simulink model "SOC_SOP_SOE_Estimator_prev"  (R2022b)
settings: Solver=VariableStepAuto  StartTime=0.0  StopTime=10.0  RelTol=1e-3
values from neighbouring files (symbols this model uses):
  C1_Matrix = 422.2404285437554 832.53586872460221 593.83691968900087 100.00008052662714 100.0001060028228 100.00352207851405 573.68336177620586 595.79755617901333 100.00046144734698 100.00010895024188 100.00001099617816 100.00006837618552 691.48671856868566 2134.4373901996432 816.34740544716044 806.77260368332577 100.0467458146305 598.37385117856434 100.00076319616421 859.37820132571676 896.36317538528124 1484    [Estimators_Dictionary.sldd]
  C2_Matrix = 1869.0199173311939 2837.236592228945 2101.4831882408225 1494.0038217573228 1387.7964069745447 1517.4535489073862 2616.2107406796117 2389.8139537375896 1452.8919060078656 1228.7968116693385 1198.856242336575 1171.693964913431 6721.2581904188037 1000.0000000113553 9531.2637756330168 5076.9051378834283 1199.7174655557417 1384.2253611332994 1210.6925685743531 5536.2724577262752 3310.8601470778594 4071    [Estimators_Dictionary.sldd]
  C3_Matrix = 10000.000413012229 10000.437423538908 10000.000000002954 999999.99836905929 999999.99999998079 10000.000000003132 10006.050761940998 10005.494579451251 10000.00000000291 999999.999999997 999999.99999999709 999999.99999999709 10000.206379215075 999999.999999997 10000.0000221827 10000.008256352026 25318.524233270309 999999.99999986857 999999.99999999709 33014.106269942291 10000.002694208375 10000.00    [Estimators_Dictionary.sldd]
  Capacity_Vec : value not decoded    [Estimators_Dictionary.sldd]
  Current_Vec : value not decoded    [Estimators_Dictionary.sldd]
  Initial_Covariance : value not decoded    [Estimators_Dictionary.sldd]
  L_SOP = 10.0    [Estimators_Dictionary.sldd]
  MaxChargeCurrent = -4.5    [Estimators_Dictionary.sldd]
  MaxDischargeCurrent = 13.5    [Estimators_Dictionary.sldd]
  Measurement_Noise_Covariance : value not decoded    [Estimators_Dictionary.sldd]
  NumberSt = 4.0    [Estimators_Dictionary.sldd]
  NumModules = 1.0    [Global_Parameters.sldd]
  NumParallel = 30.0    [Global_Parameters.sldd]
  NumSeries = 24.0    [Global_Parameters.sldd]
  OCV_25 = 2.499931353 2.660173565 2.770290801 2.849668545 2.910864288 2.961377818 3.004426237 3.041700228 3.074206823 3.103359053 3.130289569 3.156365364 3.182882947 3.209913924 3.23738746 3.264399583 3.29032752 3.314243172 3.336274664 3.356562434 3.375508383 3.393471938 3.410420203 3.425459892 3.444565547 3.460488492 3.470240307 3.477937034 3.484868617 3.491737023 3.49969269 3.561668176 3.613859701 3.66247    [Estimators_Dictionary.sldd]
  OCV_Matrix = 2.499880511 2.757887899 2.885852779 2.958886734 3.012482188 3.054053996 3.088246035 3.118484978 3.146762309 3.174638012 3.202260862 3.229457219 3.25550064 3.2799103 3.302460407 3.323174742 3.342372966 3.36043721 3.377577579 3.393845327 3.409287366 3.424345095 3.438835902 3.451705646 3.462748292 3.471979517 3.479948585 3.487316883 3.494719929 3.502771519 3.512228835 3.565792216 3.611361646 3.654868    [Estimators_Dictionary.sldd]
  Process_Noise_Covariance : value not decoded    [Estimators_Dictionary.sldd]
  R0_Matrix = 0.078 0.065280058 0.057635214 0.051424984 0.047235164 0.045274346 0.044600944 0.044414272 0.043883424 0.043849968 0.043505816 0.043376214 0.042951864 0.042984622 0.04246783 0.042081824 0.04225864 0.042254038 0.042812396 0.044036376 0.046360714 0.04 0.027933632 0.02654818 0.0250776 0.024521118 0.02407035 0.023664778 0.023539386 0.023690548 0.023919438 0.023613406 0.023919438 0.023462652 0.023664778    [Estimators_Dictionary.sldd]
  R1_Matrix = 0.0088889584036008756 0.011132450225251986 0.0047020868736295475 0.0038328697373028187 0.0040332105595120874 0.0042459601469587993 0.0079556549223052976 0.0077202921614856973 0.0042458367238840319 0.0037380352668936129 0.0039024749524341363 0.0039171117297991413 0.011740686313090084 0.019999999846677257 0.016223479832535404 0.012377879169958896 0.0036112899599241629 0.0044757607076317636 0.0037164    [Estimators_Dictionary.sldd]
  R2_Matrix = 0.019999839352755313 0.018530158856651584 0.019999999999991039 0.019999999999999653 0.019094577060873957 0.019999999999999653 0.017574853989291029 0.018122428670813852 0.01999999999999965 0.017630542321676212 0.018068015705526037 0.018465022507068402 0.005950765066923343 0.0091611667859414717 0.0094260137994600333 0.010899029961443308 0.019999999999999508 0.019999999993878602 0.018482036338747981    [Estimators_Dictionary.sldd]
  R3_Matrix = 0.011000556558775975 0.0057135937221727282 0.0099840161409517954 0.0010000000000003474 0.0010000000000003476 0.0011277504341113288 0.002355571622354306 0.0020545810808267474 0.0011567518791196808 0.00100000000000035 0.0010000000000003485 0.0010000000000003491 0.0045246675537304517 0.0010000000004847253 0.0058172911331956572 0.0046897007611929825 0.003722001496194627 0.0010000000001368907 0.0010000    [Estimators_Dictionary.sldd]
  RC_SOC_Vec : value not decoded    [Estimators_Dictionary.sldd]
  SOC_Max = 1.0    [Estimators_Dictionary.sldd]
  SOC_Min = 0.0    [Estimators_Dictionary.sldd]
  SOC_Vec1 : value not decoded    [Estimators_Dictionary.sldd]
  SOC_Vec2 = 0.0426283206867574 0.0904968112442659 0.138364796472968 0.186232899174877 0.234100725864356 0.281969477464203 0.329837548126425 0.37770754411239 0.425577249630283 0.473445315109007 0.52131352299741 0.569182352268543 0.617052114517866 0.664920478266386 0.712789145362285 0.760657112801272 0.808525199586941 0.856393952315712 0.904262172378725 0.952130333891273 1.0    [Estimators_Dictionary.sldd]
  SOH_Vec : value not decoded    [Estimators_Dictionary.sldd]
  Temperature_Vec : value not decoded    [Estimators_Dictionary.sldd]
  Ts = 0.01    [Global_Parameters.sldd]
  Ts_SOP = 15.0    [Estimators_Dictionary.sldd]
  V1_Max = 0.01    [Estimators_Dictionary.sldd]
  V1_Min = -0.01    [Estimators_Dictionary.sldd]
  V2_Max = 0.01    [Estimators_Dictionary.sldd]
  V2_Min = -0.01    [Estimators_Dictionary.sldd]
  V3_Max = 0.01    [Estimators_Dictionary.sldd]
  V3_Min = -0.01    [Estimators_Dictionary.sldd]
  Vmax = 4.1    [Global_Parameters.sldd]
  Vmin = 3.0    [Global_Parameters.sldd]
settings Model: DataDictionary=Estimators_Dictionary.sldd  Creator=japerez  LastModifiedBy=CMARTINEZ
settings DebuggingCC: ParameterPrecisionLossMsg=none

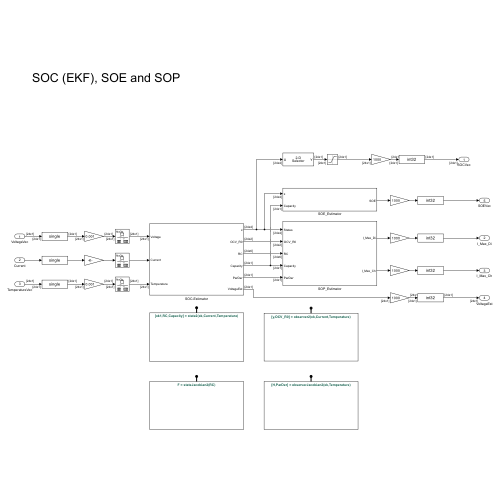
[thumbnail: Simulink's stored preview of the top-level diagram]
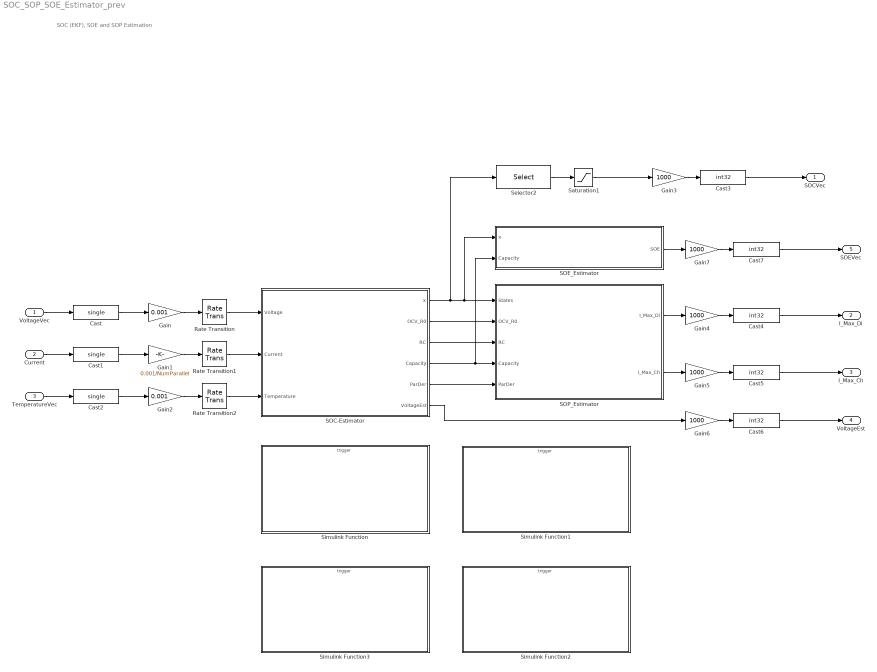
== system SOC_SOP_SOE_Estimator_prev ==
  note: SOC (EKF), SOE and SOP Estimation
  VoltageVec : Inport  OutDataTypeStr=int32  PortDimensions=[NumSeries*NumModules,1]
  Current : Inport  Port=2  OutDataTypeStr=int32  PortDimensions=1
  TemperatureVec : Inport  Port=3  OutDataTypeStr=int32  PortDimensions=[NumSeries*NumModules,1]
  Cast : DataTypeConversion  OutDataTypeStr=single  SaturateOnIntegerOverflow=off  RndMeth=Floor
  Cast1 : DataTypeConversion  OutDataTypeStr=single  SaturateOnIntegerOverflow=off  RndMeth=Floor
  Cast2 : DataTypeConversion  OutDataTypeStr=single  SaturateOnIntegerOverflow=off  RndMeth=Floor
  Cast{3..7} (5 alike) : DataTypeConversion  OutDataTypeStr=int32  SaturateOnIntegerOverflow=off  RndMeth=Floor
  Gain : Gain  Gain=0.001
  Gain1 : Gain  Gain=0.001/NumParallel
  Gain2 : Gain  Gain=0.001
  Gain{3..7} (5 alike) : Gain  Gain=1000
  Rate Transition : RateTransition  Integrity=off  OutPortSampleTime=Ts
  Rate Transition1 : RateTransition  Integrity=off  OutPortSampleTime=Ts
  Rate Transition2 : RateTransition  Integrity=off  OutPortSampleTime=Ts
  SOC-Estimator : Subsystem
  SOE_Estimator : Subsystem
  SOP_Estimator : Subsystem
  Saturation1 : Saturate  UpperLimit=1  LowerLimit=0
  Selector2 : Selector  NumberOfDimensions=2  InputPortWidth=24  IndexOptions=Select all,Index vector (dialog)  Indices=1,1  OutputSizes=1,1
  Simulink Function : Subsystem  TreatAsAtomicUnit=on
  Simulink Function1 : Subsystem  TreatAsAtomicUnit=on
  Simulink Function2 : Subsystem  TreatAsAtomicUnit=on
  Simulink Function3 : Subsystem  TreatAsAtomicUnit=on
  SOCVec : Outport  OutDataTypeStr=int32  PortDimensions=[NumSeries*NumModules,1]
  I_Max_Di : Outport  Port=2  OutDataTypeStr=int32  PortDimensions=1
  I_Max_Ch : Outport  Port=3  OutDataTypeStr=int32  PortDimensions=1
  VoltageEst : Outport  Port=4  OutDataTypeStr=int32  PortDimensions=[NumSeries*NumModules,1]
  SOEVec : Outport  Port=5
  wires:
  Gain/1 -> Rate Transition/1
  Rate Transition2/1 -> SOC-Estimator/3(Temperature)
  Gain1/1 -> Rate Transition1/1
  Selector2/1 -> Saturation1/1
  VoltageVec/1 -> Cast/1
  Current/1 -> Cast1/1
  TemperatureVec/1 -> Cast2/1
  Cast/1 -> Gain/1
  Cast1/1 -> Gain1/1
  Cast2/1 -> Gain2/1
  Gain2/1 -> Rate Transition2/1
  Gain3/1 -> Cast3/1
  Saturation1/1 -> Gain3/1
  SOC-Estimator/1(x) -> SOE_Estimator/1(x), SOP_Estimator/1(States), Selector2/1
  SOC-Estimator/2(OCV_R0) -> SOP_Estimator/2(OCV_R0)
  SOC-Estimator/3(RC) -> SOP_Estimator/3(RC)
  SOC-Estimator/4(Capacity) -> SOE_Estimator/2(Capacity), SOP_Estimator/4(Capacity)
  SOC-Estimator/5(ParDer) -> SOP_Estimator/5(ParDer)
  Gain4/1 -> Cast4/1
  SOP_Estimator/1(I_Max_Di) -> Gain4/1
  Gain5/1 -> Cast5/1
  SOP_Estimator/2(I_Max_Ch) -> Gain5/1
  Gain6/1 -> Cast6/1
  SOC-Estimator/6(VoltageEst) -> Gain6/1
  Rate Transition1/1 -> SOC-Estimator/2(Current)
  Rate Transition/1 -> SOC-Estimator/1(Voltage)
  Cast3/1 -> SOCVec/1
  Cast4/1 -> I_Max_Di/1
  Cast5/1 -> I_Max_Ch/1
  Cast6/1 -> VoltageEst/1
  SOE_Estimator/1(SOE) -> Gain7/1
  Gain7/1 -> Cast7/1
  Cast7/1 -> SOEVec/1

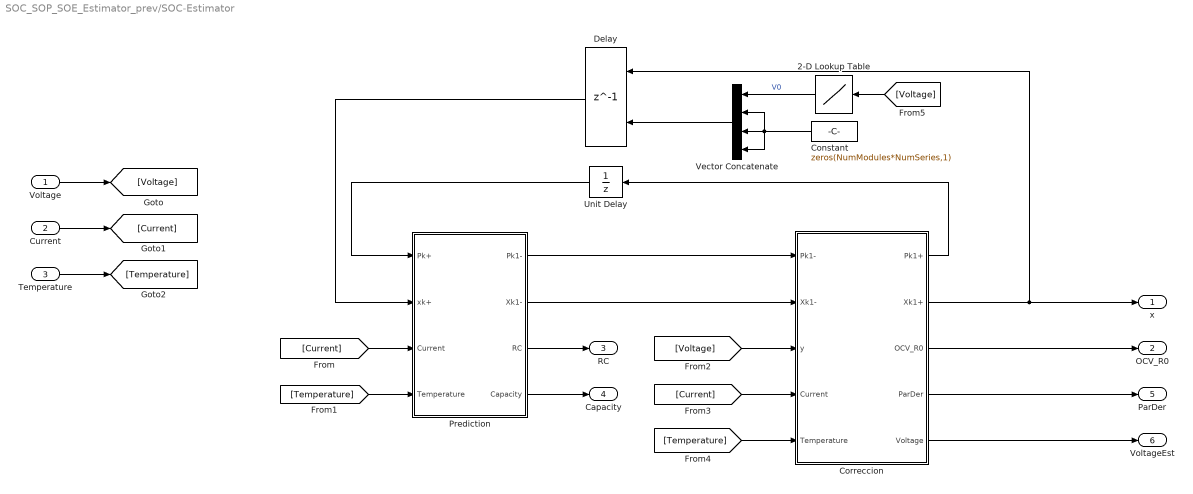
== system SOC_SOP_SOE_Estimator_prev/SOC-Estimator ==
  Voltage : Inport
  Current : Inport  Port=2
  Temperature : Inport  Port=3
  2-D Lookup Table : Lookup_n-D  NumberOfTableDimensions=1  BreakpointsForDimension1=OCV_25  BreakpointsForDimension2=Temperature_Vec  BreakpointsForDimension3=SOH_Vec  Table=SOC_Vec1  ExtrapMethod=Clip  InternalRulePriority=Speed  RndMeth=Simplest
  Constant : Constant  Value=zeros(NumModules*NumSeries,1)  OutDataTypeStr=single
  Correccion : Subsystem
  Delay : Delay  DelayLength=1  InitialConditionSource=Input port
      settings: InputPortMap=u0,p4
  Prediction : Subsystem
  Unit Delay : UnitDelay  InitialCondition=Initial_Covariance.*ones(NumModules*NumSeries,NumberSt)  SampleTime=Ts  HasFrameUpgradeWarning=on
  Vector Concatenate : Concatenate  NumInputs=4  Mode=Multidimensional array  ConcatenateDimension=2
  x : Outport
  OCV_R0 : Outport  Port=2
  RC : Outport  Port=3
  Capacity : Outport  Port=4
  ParDer : Outport  Port=5
  VoltageEst : Outport  Port=6
  wires:
  [Current] -> Prediction/3(Current)
  [Temperature] -> Prediction/4(Temperature)
  Temperature/1 -> [Temperature]
  Correccion/1(Pk1+) -> Unit Delay/1
  Prediction/1(Pk1-) -> Correccion/1(Pk1-)
  Prediction/2(Xk1-) -> Correccion/2(Xk1-)
  Correccion/2(Xk1+) -> Delay/1, x/1
  [Voltage] -> Correccion/3(y)
  Voltage/1 -> [Voltage]
  Current/1 -> [Current]
  Unit Delay/1 -> Prediction/1(Pk+)
  [Temperature] -> Correccion/5(Temperature)
  [Current] -> Correccion/4(Current)
  Correccion/3(OCV_R0) -> OCV_R0/1
  Delay/1 -> Prediction/2(xk+)
  Prediction/3(RC) -> RC/1
  Prediction/4(Capacity) -> Capacity/1
  Correccion/4(ParDer) -> ParDer/1
  Correccion/5(Voltage) -> VoltageEst/1
  Constant/1 -> Vector Concatenate/2, Vector Concatenate/3, Vector Concatenate/4
  2-D Lookup Table/1 -> Vector Concatenate/1  "V0"
  Vector Concatenate/1 -> Delay/2
  [Voltage] -> 2-D Lookup Table/1

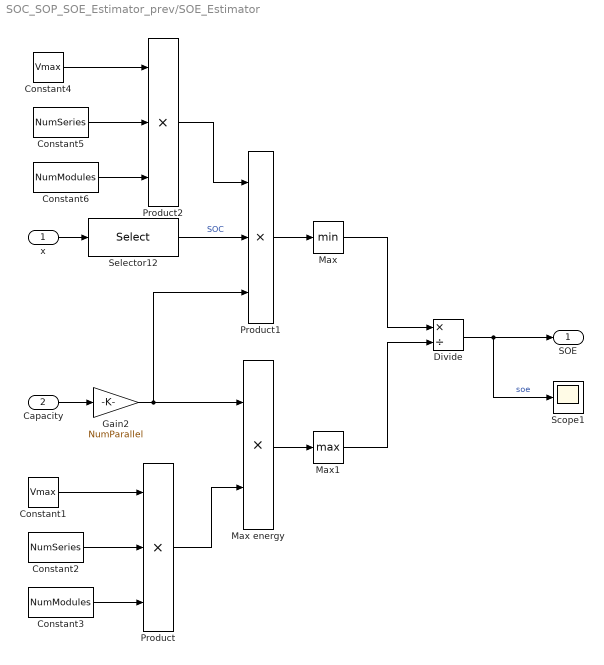
== system SOC_SOP_SOE_Estimator_prev/SOE_Estimator ==
  x : Inport
  Capacity : Inport  Port=2
  Constant1 : Constant  Value=Vmax
  Constant2 : Constant  Value=NumSeries
  Constant3 : Constant  Value=NumModules
  Constant4 : Constant  Value=Vmax
  Constant5 : Constant  Value=NumSeries
  Constant6 : Constant  Value=NumModules
  Divide : Product  Inputs=*/
  Gain2 : Gain  Gain=NumParallel
  Max : MinMax
  Max energy : Product
  Max1 : MinMax  Function=max
  Product : Product  Inputs=3
  Product1 : Product  Inputs=3
  Product2 : Product  Inputs=3
  Scope1 : Scope
  Selector12 : Selector  NumberOfDimensions=2  InputPortWidth=24  IndexOptions=Select all,Index vector (dialog)  Indices=1,1  OutputSizes=1,1
  SOE : Outport  OutDataTypeStr=single
  wires:
  x/1 -> Selector12/1
  Constant1/1 -> Product/1
  Constant2/1 -> Product/2
  Capacity/1 -> Gain2/1
  Product/1 -> Max energy/2
  Max/1 -> Divide/1
  Max1/1 -> Divide/2
  Divide/1 -> SOE/1, Scope1/1  "soe"
  Product1/1 -> Max/1
  Max energy/1 -> Max1/1
  Constant3/1 -> Product/3
  Selector12/1 -> Product1/2  "SOC"
  Constant6/1 -> Product2/3
  Constant5/1 -> Product2/2
  Constant4/1 -> Product2/1
  Product2/1 -> Product1/1
  Gain2/1 -> Product1/3, Max energy/1

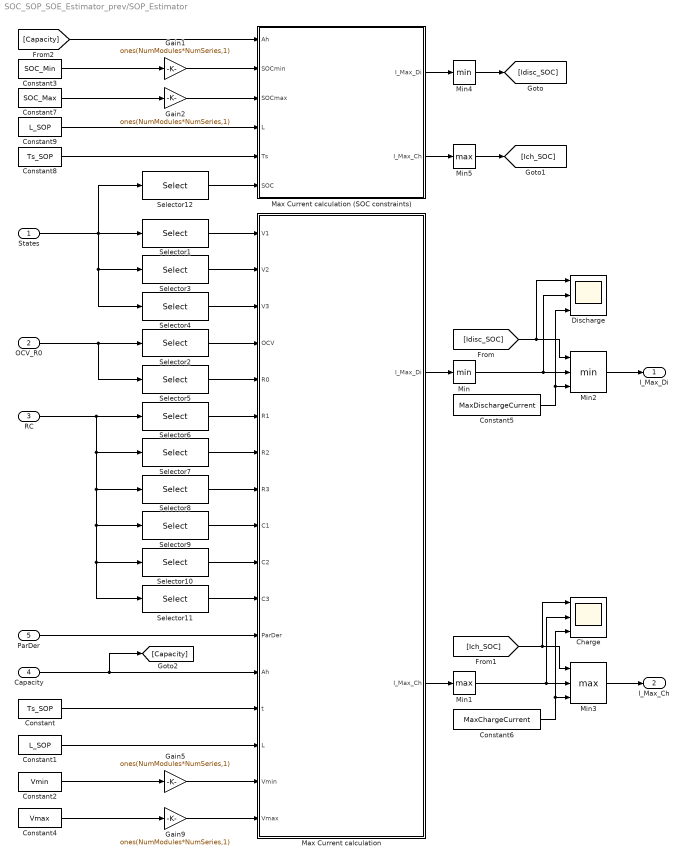
== system SOC_SOP_SOE_Estimator_prev/SOP_Estimator ==
  States : Inport  OutDataTypeStr=single  PortDimensions=[NumModules*NumSeries,NumberSt]
  OCV_R0 : Inport  Port=2  OutDataTypeStr=single  PortDimensions=[NumModules*NumSeries,2]
  RC : Inport  Port=3  OutDataTypeStr=single  PortDimensions=[NumModules*NumSeries,6]
  Capacity : Inport  Port=4  OutDataTypeStr=single  PortDimensions=[NumModules*NumSeries,1]
  ParDer : Inport  Port=5  OutDataTypeStr=single  PortDimensions=[NumModules*NumSeries,1]
  Charge : Scope  NumInputPorts=3
  Constant : Constant  Value=Ts_SOP
  Constant1 : Constant  Value=L_SOP
  Constant2 : Constant  Value=Vmin  OutDataTypeStr=single
  Constant3 : Constant  Value=SOC_Min  OutDataTypeStr=single
  Constant4 : Constant  Value=Vmax  OutDataTypeStr=single
  Constant5 : Constant  Value=MaxDischargeCurrent
  Constant6 : Constant  Value=MaxChargeCurrent
  Constant7 : Constant  Value=SOC_Max  OutDataTypeStr=single
  Constant8 : Constant  Value=Ts_SOP
  Constant9 : Constant  Value=L_SOP
  Discharge : Scope  NumInputPorts=3
  Gain{1..2,5,9} (4 alike) : Gain  Gain=ones(NumModules*NumSeries,1)  ParamDataTypeStr=single  OutDataTypeStr=single
  Max Current calculation : MATLAB Function  TreatAsAtomicUnit=on
  Max Current calculation (SOC constraints) : MATLAB Function  TreatAsAtomicUnit=on
  Min : MinMax
  Min1 : MinMax  Function=max
  Min2 : MinMax  Inputs=3
  Min3 : MinMax  Function=max  Inputs=3
  Min4 : MinMax
  Min5 : MinMax  Function=max
  Selector1 : Selector  NumberOfDimensions=2  InputPortWidth=24  IndexOptions=Select all,Index vector (dialog)  Indices=1,2  OutputSizes=1,1
  Selector10 : Selector  NumberOfDimensions=2  InputPortWidth=24  IndexOptions=Select all,Index vector (dialog)  Indices=1,5  OutputSizes=1,1
  Selector11 : Selector  NumberOfDimensions=2  InputPortWidth=24  IndexOptions=Select all,Index vector (dialog)  Indices=1,6  OutputSizes=1,1
  Selector12 : Selector  NumberOfDimensions=2  InputPortWidth=24  IndexOptions=Select all,Index vector (dialog)  Indices=1,1  OutputSizes=1,1
  Selector2 : Selector  NumberOfDimensions=2  InputPortWidth=24  IndexOptions=Select all,Index vector (dialog)  Indices=1,1  OutputSizes=1,1
  Selector3 : Selector  NumberOfDimensions=2  InputPortWidth=24  IndexOptions=Select all,Index vector (dialog)  Indices=1,3  OutputSizes=1,1
  Selector4 : Selector  NumberOfDimensions=2  InputPortWidth=24  IndexOptions=Select all,Index vector (dialog)  Indices=1,4  OutputSizes=1,1
  Selector5 : Selector  NumberOfDimensions=2  InputPortWidth=24  IndexOptions=Select all,Index vector (dialog)  Indices=1,2  OutputSizes=1,1
  Selector6 : Selector  NumberOfDimensions=2  InputPortWidth=24  IndexOptions=Select all,Index vector (dialog)  Indices=1,1  OutputSizes=1,1
  Selector7 : Selector  NumberOfDimensions=2  InputPortWidth=24  IndexOptions=Select all,Index vector (dialog)  Indices=1,2  OutputSizes=1,1
  Selector8 : Selector  NumberOfDimensions=2  InputPortWidth=24  IndexOptions=Select all,Index vector (dialog)  Indices=1,3  OutputSizes=1,1
  Selector9 : Selector  NumberOfDimensions=2  InputPortWidth=24  IndexOptions=Select all,Index vector (dialog)  Indices=1,4  OutputSizes=1,1
  I_Max_Di : Outport  OutDataTypeStr=single  PortDimensions=1
  I_Max_Ch : Outport  Port=2  OutDataTypeStr=single  PortDimensions=1
  wires:
  Selector1/1 -> Max Current calculation/1(V1)
  Selector5/1 -> Max Current calculation/5(R0)
  Constant2/1 -> Gain5/1
  Max Current calculation/2(I_Max_Ch) -> Min1/1
  Min2/1 -> I_Max_Di/1
  Max Current calculation/1(I_Max_Di) -> Min/1
  Constant4/1 -> Gain9/1
  OCV_R0/1 -> Selector5/1, Selector2/1
  Gain5/1 -> Max Current calculation/16(Vmin)
  Capacity/1 -> [Capacity], Max Current calculation/13(Ah)
  Selector3/1 -> Max Current calculation/2(V2)
  Min3/1 -> I_Max_Ch/1
  RC/1 -> Selector11/1, Selector10/1, Selector9/1, Selector8/1, Selector7/1, Selector6/1
  Selector2/1 -> Max Current calculation/4(OCV)
  Selector6/1 -> Max Current calculation/6(R1)
  Selector11/1 -> Max Current calculation/11(C3)
  Selector10/1 -> Max Current calculation/10(C2)
  Selector9/1 -> Max Current calculation/9(C1)
  ParDer/1 -> Max Current calculation/12(ParDer)
  Selector8/1 -> Max Current calculation/8(R3)
  Selector7/1 -> Max Current calculation/7(R2)
  Selector4/1 -> Max Current calculation/3(V3)
  Constant1/1 -> Max Current calculation/15(L)
  Gain9/1 -> Max Current calculation/17(Vmax)
  Constant3/1 -> Gain1/1
  States/1 -> Selector12/1, Selector4/1, Selector3/1, Selector1/1
  Constant7/1 -> Gain2/1
  Selector12/1 -> Max Current calculation (SOC constraints)/6(SOC)
  Gain2/1 -> Max Current calculation (SOC constraints)/3(SOCmax)
  Gain1/1 -> Max Current calculation (SOC constraints)/2(SOCmin)
  Max Current calculation (SOC constraints)/1(I_Max_Di) -> Min4/1
  Max Current calculation (SOC constraints)/2(I_Max_Ch) -> Min5/1
  Min4/1 -> [Idisc_SOC]
  Min5/1 -> [Ich_SOC]
  Min/1 -> Discharge/2, Min2/2
  [Idisc_SOC] -> Discharge/1, Min2/1
  Constant6/1 -> Min3/3, Charge/3
  [Ich_SOC] -> Charge/1, Min3/1
  [Capacity] -> Max Current calculation (SOC constraints)/1(Ah)
  Min1/1 -> Charge/2, Min3/2
  Constant5/1 -> Discharge/3, Min2/3
  Constant9/1 -> Max Current calculation (SOC constraints)/4(L)
  Constant8/1 -> Max Current calculation (SOC constraints)/5(Ts)
  Constant/1 -> Max Current calculation/14(t)

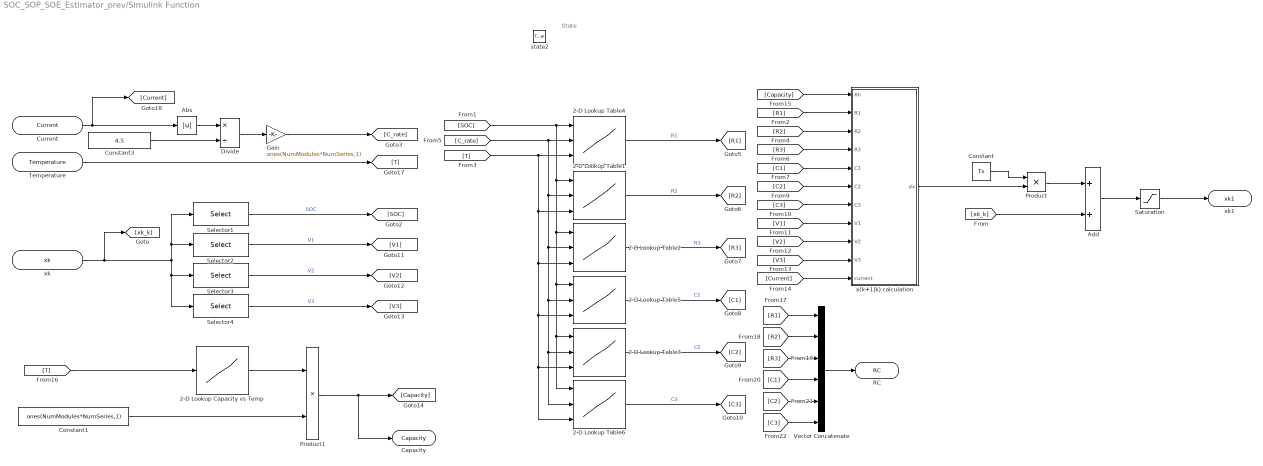
== system SOC_SOP_SOE_Estimator_prev/Simulink Function ==
  note: State
  state2 : TriggerPort  TriggerType=function-call  IsSimulinkFunction=on  FunctionName=state2  FunctionVisibility=scoped  VariantControl=(inherit)
  2-D Lookup Capacity vs Temp : Lookup_n-D  NumberOfTableDimensions=1  BreakpointsForDimension1=Temperature_Vec  BreakpointsForDimension2=Current_Vec  BreakpointsForDimension3=Temperature_Vec  BreakpointsForDimension4=SOH_Vec  Table=Capacity_Vec  InternalRulePriority=Speed  RndMeth=Simplest
  2-D Lookup Table1 : Lookup_n-D  NumberOfTableDimensions=3  BreakpointsForDimension1=RC_SOC_Vec  BreakpointsForDimension2=Current_Vec  BreakpointsForDimension3=Temperature_Vec  BreakpointsForDimension4=SOH_Vec  Table=R2_Matrix  ExtrapMethod=Clip  InternalRulePriority=Speed  RndMeth=Simplest
      settings: InputPortMap=u0,u1,u2
  2-D Lookup Table2 : Lookup_n-D  NumberOfTableDimensions=3  BreakpointsForDimension1=RC_SOC_Vec  BreakpointsForDimension2=Current_Vec  BreakpointsForDimension3=Temperature_Vec  BreakpointsForDimension4=SOH_Vec  Table=R3_Matrix  ExtrapMethod=Clip  InternalRulePriority=Speed  RndMeth=Simplest
      settings: InputPortMap=u0,u1,u2
  2-D Lookup Table3 : Lookup_n-D  NumberOfTableDimensions=3  BreakpointsForDimension1=RC_SOC_Vec  BreakpointsForDimension2=Current_Vec  BreakpointsForDimension3=Temperature_Vec  BreakpointsForDimension4=SOH_Vec  Table=C2_Matrix  ExtrapMethod=Clip  InternalRulePriority=Speed  RndMeth=Simplest
      settings: InputPortMap=u0,u1,u2
  2-D Lookup Table4 : Lookup_n-D  NumberOfTableDimensions=3  BreakpointsForDimension1=RC_SOC_Vec  BreakpointsForDimension2=Current_Vec  BreakpointsForDimension3=Temperature_Vec  BreakpointsForDimension4=SOH_Vec  Table=R1_Matrix  ExtrapMethod=Clip  InternalRulePriority=Speed  RndMeth=Simplest
      settings: InputPortMap=u0,u1,u2
  2-D Lookup Table5 : Lookup_n-D  NumberOfTableDimensions=3  BreakpointsForDimension1=RC_SOC_Vec  BreakpointsForDimension2=Current_Vec  BreakpointsForDimension3=Temperature_Vec  BreakpointsForDimension4=SOH_Vec  Table=C1_Matrix  ExtrapMethod=Clip  InternalRulePriority=Speed  RndMeth=Simplest
      settings: InputPortMap=u0,u1,u2
  2-D Lookup Table6 : Lookup_n-D  NumberOfTableDimensions=3  BreakpointsForDimension1=RC_SOC_Vec  BreakpointsForDimension2=Current_Vec  BreakpointsForDimension3=Temperature_Vec  BreakpointsForDimension4=SOH_Vec  Table=C3_Matrix  ExtrapMethod=Clip  InternalRulePriority=Speed  RndMeth=Simplest
      settings: InputPortMap=u0,u1,u2
  Abs : Abs  SaturateOnIntegerOverflow=off
  Add : Sum  AccumDataTypeStr=single  OutDataTypeStr=single
  Constant : Constant  Value=Ts
  Constant1 : Constant  Value=ones(NumModules*NumSeries,1)  OutDataTypeStr=single
  Constant3 : Constant  Value=4.5  OutDataTypeStr=single
  Divide : Product  Inputs=*/  OutDataTypeStr=single
  Gain : Gain  Gain=ones(NumModules*NumSeries,1)  ParamDataTypeStr=single  OutDataTypeStr=single
  Product : Product
  Product1 : Product  OutDataTypeStr=single
  Saturation : Saturate  UpperLimit=[SOC_Max,V1_Max,V2_Max,V3_Max].*ones(NumModules*NumSeries,NumberSt)  LowerLimit=[SOC_Min,V1_Min,V2_Min,V3_Min].*ones(NumModules*NumSeries,NumberSt)  OutDataTypeStr=single
  Selector1 : Selector  NumberOfDimensions=2  InputPortWidth=24  IndexOptions=Select all,Index vector (dialog)  Indices=1,1  OutputSizes=1,1
  Selector2 : Selector  NumberOfDimensions=2  InputPortWidth=24  IndexOptions=Select all,Index vector (dialog)  Indices=2,2  OutputSizes=1,1
  Selector3 : Selector  NumberOfDimensions=2  InputPortWidth=24  IndexOptions=Select all,Index vector (dialog)  Indices=3,3  OutputSizes=1,1
  Selector4 : Selector  NumberOfDimensions=2  InputPortWidth=24  IndexOptions=Select all,Index vector (dialog)  Indices=4,4  OutputSizes=1,1
  Vector Concatenate : Concatenate  NumInputs=6  Mode=Multidimensional array  ConcatenateDimension=2
  x(k+1|k) calculation : MATLAB Function  TreatAsAtomicUnit=on
  xk : ArgIn  DisableCoverage=on  OutDataTypeStr=single  PortDimensions=[NumSeries*NumModules,NumberSt]  ArgumentName=xk
  Current : ArgIn  DisableCoverage=on  Port=2  OutDataTypeStr=single  ArgumentName=Current
  Temperature : ArgIn  DisableCoverage=on  Port=3  OutDataTypeStr=single  PortDimensions=[NumSeries*NumModules,1]  ArgumentName=Temperature
  xk1 : ArgOut  DisableCoverage=on  OutDataTypeStr=single  PortDimensions=[NumModules*NumSeries,NumberSt]  ArgumentName=xk1
  RC : ArgOut  DisableCoverage=on  Port=2  OutDataTypeStr=single  PortDimensions=[NumModules*NumSeries,6]  ArgumentName=RC
  Capacity : ArgOut  DisableCoverage=on  Port=3  OutDataTypeStr=single  PortDimensions=[NumModules*NumSeries,1]  ArgumentName=Capacity
  wires:
  Divide/1 -> Gain/1
  Constant3/1 -> Divide/2
  Current/1 -> Abs/1, [Current]
  [Current] -> x(k+1|k) calculation/11(current)
  [V3] -> x(k+1|k) calculation/10(V3)
  [V2] -> x(k+1|k) calculation/9(V2)
  [V1] -> x(k+1|k) calculation/8(V1)
  Selector4/1 -> [V3]  "V3"
  Selector3/1 -> [V2]  "V2"
  Selector2/1 -> [V1]  "V1"
  [C3] -> x(k+1|k) calculation/7(C3)
  [C2] -> x(k+1|k) calculation/6(C2)
  [C1] -> x(k+1|k) calculation/5(C1)
  [R3] -> x(k+1|k) calculation/4(R3)
  [R2] -> x(k+1|k) calculation/3(R2)
  [R1] -> x(k+1|k) calculation/2(R1)
  Selector1/1 -> [SOC]  "SOC"
  2-D Lookup Table1/1 -> [R2]  "R2"
  2-D Lookup Table2/1 -> [R3]  "R3"
  2-D Lookup Table5/1 -> [C1]  "C1"
  2-D Lookup Table3/1 -> [C2]  "C2"
  2-D Lookup Table6/1 -> [C3]  "C3"
  2-D Lookup Table4/1 -> [R1]  "R1"
  Add/1 -> Saturation/1
  xk/1 -> Selector3/1, Selector4/1, Selector2/1, Selector1/1, [xk_k]
  [Capacity] -> x(k+1|k) calculation/1(Ah)
  2-D Lookup Capacity vs Temp/1 -> Product1/1
  [T] -> 2-D Lookup Capacity vs Temp/1
  Temperature/1 -> [T]
  Vector Concatenate/1 -> RC/1
  [R1] -> Vector Concatenate/1
  [R2] -> Vector Concatenate/2
  [R3] -> Vector Concatenate/3
  [C1] -> Vector Concatenate/4
  [C2] -> Vector Concatenate/5
  [C3] -> Vector Concatenate/6
  Saturation/1 -> xk1/1
  Gain/1 -> [C_rate]
  Constant1/1 -> Product1/2
  [SOC] -> 2-D Lookup Table1/1, 2-D Lookup Table2/1, 2-D Lookup Table5/1, 2-D Lookup Table6/1, 2-D Lookup Table3/1, 2-D Lookup Table4/1
  [C_rate] -> 2-D Lookup Table1/2, 2-D Lookup Table2/2, 2-D Lookup Table5/2, 2-D Lookup Table6/2, 2-D Lookup Table3/2, 2-D Lookup Table4/2
  [T] -> 2-D Lookup Table1/3, 2-D Lookup Table2/3, 2-D Lookup Table5/3, 2-D Lookup Table6/3, 2-D Lookup Table3/3, 2-D Lookup Table4/3
  Product1/1 -> Capacity/1, [Capacity]
  Abs/1 -> Divide/1
  [xk_k] -> Add/2
  x(k+1|k) calculation/1(dx) -> Product/2
  Product/1 -> Add/1
  Constant/1 -> Product/1

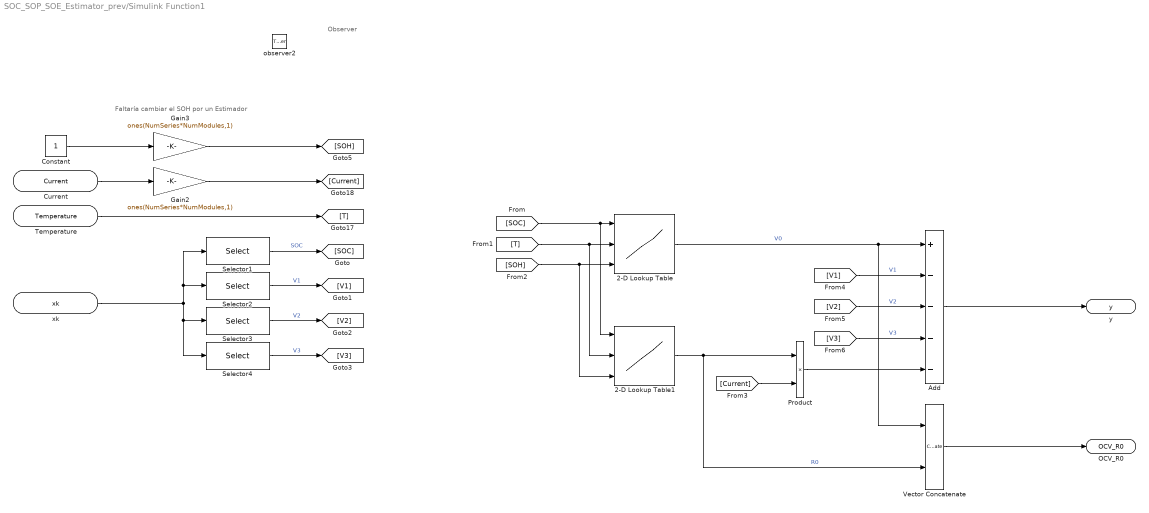
== system SOC_SOP_SOE_Estimator_prev/Simulink Function1 ==
  note: Faltaría cambiar el SOH por un Estimador
  note: Observer
  observer2 : TriggerPort  TriggerType=function-call  IsSimulinkFunction=on  FunctionName=observer2  FunctionVisibility=scoped  VariantControl=(inherit)
  2-D Lookup Table : Lookup_n-D  NumberOfTableDimensions=3  BreakpointsForDimension1=SOC_Vec1  BreakpointsForDimension2=Temperature_Vec  BreakpointsForDimension3=SOH_Vec  Table=OCV_Matrix  ExtrapMethod=Clip  InternalRulePriority=Speed  RndMeth=Simplest
      settings: InputPortMap=u0,u1,u2
  2-D Lookup Table1 : Lookup_n-D  NumberOfTableDimensions=3  BreakpointsForDimension1=SOC_Vec2  BreakpointsForDimension2=Temperature_Vec  BreakpointsForDimension3=SOH_Vec  Table=R0_Matrix  ExtrapMethod=Clip  InternalRulePriority=Speed  RndMeth=Simplest
      settings: InputPortMap=u0,u1,u2
  Add : Sum  Inputs=+----
  Constant : Constant  OutDataTypeStr=single
  Gain2 : Gain  Gain=ones(NumSeries*NumModules,1)
  Gain3 : Gain  Gain=ones(NumSeries*NumModules,1)
  Product : Product
  Selector1 : Selector  NumberOfDimensions=2  InputPortWidth=24  IndexOptions=Select all,Index vector (dialog)  Indices=1,1  OutputSizes=1,1
  Selector2 : Selector  NumberOfDimensions=2  InputPortWidth=24  IndexOptions=Select all,Index vector (dialog)  Indices=2,2  OutputSizes=1,1
  Selector3 : Selector  NumberOfDimensions=2  InputPortWidth=24  IndexOptions=Select all,Index vector (dialog)  Indices=3,3  OutputSizes=1,1
  Selector4 : Selector  NumberOfDimensions=2  InputPortWidth=24  IndexOptions=Select all,Index vector (dialog)  Indices=4,4  OutputSizes=1,1
  Vector Concatenate : Concatenate  Mode=Multidimensional array  ConcatenateDimension=2
  xk : ArgIn  DisableCoverage=on  OutDataTypeStr=single  PortDimensions=[NumModules*NumSeries,NumberSt]  ArgumentName=xk
  Current : ArgIn  DisableCoverage=on  Port=2  OutDataTypeStr=single  PortDimensions=[1]  ArgumentName=Current
  Temperature : ArgIn  DisableCoverage=on  Port=3  OutDataTypeStr=single  PortDimensions=[NumModules*NumSeries,1]  ArgumentName=Temperature
  y : ArgOut  DisableCoverage=on  OutDataTypeStr=single  PortDimensions=[NumModules*NumSeries,1]  ArgumentName=y
  OCV_R0 : ArgOut  DisableCoverage=on  Port=2  OutDataTypeStr=single  PortDimensions=[NumModules*NumSeries,2]  ArgumentName=OCV_R0
  wires:
  Current/1 -> Gain2/1
  [V3] -> Add/4  "V3"
  Constant/1 -> Gain3/1
  Selector4/1 -> [V3]  "V3"
  Selector3/1 -> [V2]  "V2"
  Selector2/1 -> [V1]  "V1"
  [V2] -> Add/3  "V2"
  [V1] -> Add/2  "V1"
  Selector1/1 -> [SOC]  "SOC"
  Add/1 -> y/1
  Product/1 -> Add/5
  [Current] -> Product/2
  2-D Lookup Table/1 -> Vector Concatenate/1, Add/1  "V0"
  2-D Lookup Table1/1 -> Vector Concatenate/2, Product/1  "R0"
  Temperature/1 -> [T]
  xk/1 -> Selector2/1, Selector1/1, Selector3/1, Selector4/1
  Gain3/1 -> [SOH]
  Gain2/1 -> [Current]
  [SOC] -> 2-D Lookup Table1/1, 2-D Lookup Table/1
  [T] -> 2-D Lookup Table1/2, 2-D Lookup Table/2
  [SOH] -> 2-D Lookup Table1/3, 2-D Lookup Table/3
  Vector Concatenate/1 -> OCV_R0/1

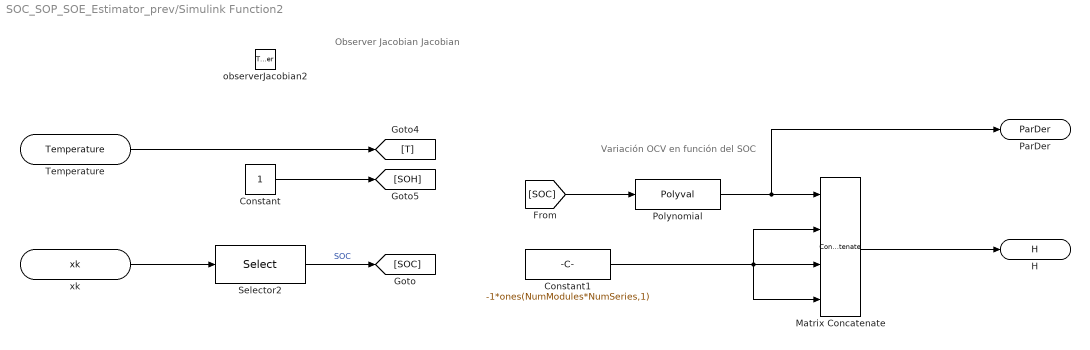
== system SOC_SOP_SOE_Estimator_prev/Simulink Function2 ==
  note: Variación OCV en función del SOC
  note: Observer Jacobian Jacobian
  observerJacobian2 : TriggerPort  TriggerType=function-call  IsSimulinkFunction=on  FunctionName=observerJacobian2  FunctionVisibility=scoped  VariantControl=(inherit)
  Constant : Constant
  Constant1 : Constant  Value=-1*ones(NumModules*NumSeries,1)  OutDataTypeStr=single
  Matrix Concatenate : Concatenate  NumInputs=4  Mode=Multidimensional array  ConcatenateDimension=2
  Polynomial : Polyval  Coefs=[-7.321*4,17.55*3,-14.72*2,5.972]
  Selector2 : Selector  NumberOfDimensions=2  InputPortWidth=24  IndexOptions=Select all,Index vector (dialog)  Indices=1,1  OutputSizes=1,1
  xk : ArgIn  DisableCoverage=on  OutDataTypeStr=single  PortDimensions=[NumModules*NumSeries,NumberSt]  ArgumentName=xk
  Temperature : ArgIn  DisableCoverage=on  Port=2  OutDataTypeStr=single  PortDimensions=[NumModules*NumSeries,1]  ArgumentName=Temperature
  H : ArgOut  DisableCoverage=on  OutDataTypeStr=single  PortDimensions=[NumModules*NumSeries,NumberSt]  ArgumentName=H
  ParDer : ArgOut  DisableCoverage=on  Port=2  OutDataTypeStr=single  PortDimensions=[NumModules*NumSeries,1]  ArgumentName=ParDer
  wires:
  xk/1 -> Selector2/1
  Matrix Concatenate/1 -> H/1
  Selector2/1 -> [SOC]  "SOC"
  Constant/1 -> [SOH]
  Temperature/1 -> [T]
  Polynomial/1 -> ParDer/1, Matrix Concatenate/1
  [SOC] -> Polynomial/1
  Constant1/1 -> Matrix Concatenate/2, Matrix Concatenate/3, Matrix Concatenate/4

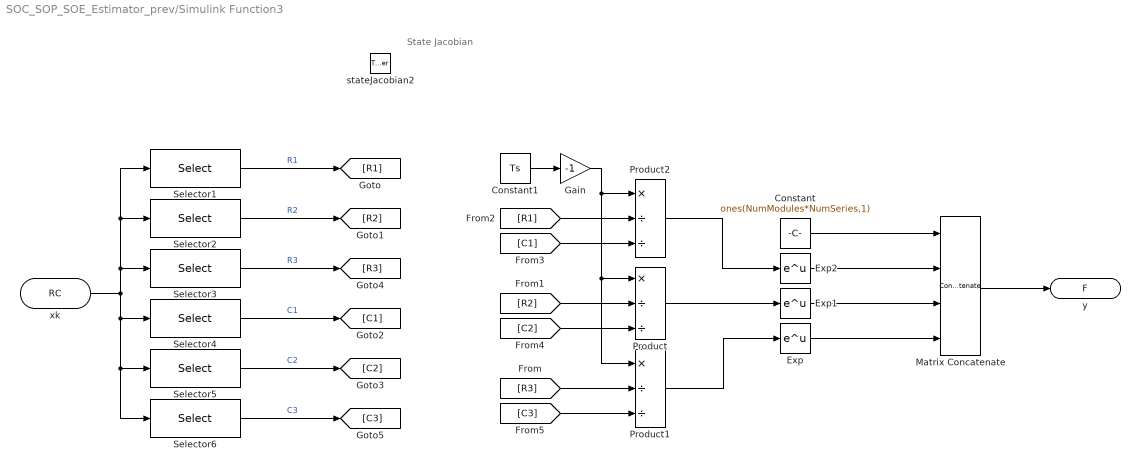
== system SOC_SOP_SOE_Estimator_prev/Simulink Function3 ==
  note: State Jacobian
  stateJacobian2 : TriggerPort  TriggerType=function-call  IsSimulinkFunction=on  FunctionName=stateJacobian2  FunctionVisibility=scoped  VariantControl=(inherit)
  Constant : Constant  Value=ones(NumModules*NumSeries,1)  OutDataTypeStr=single
  Constant1 : Constant  Value=Ts  OutDataTypeStr=single
  Exp : Math
  Exp1 : Math
  Exp2 : Math
  Gain : Gain  Gain=-1
  Matrix Concatenate : Concatenate  NumInputs=4  Mode=Multidimensional array  ConcatenateDimension=2
  Product : Product  Inputs=*//
  Product1 : Product  Inputs=*//
  Product2 : Product  Inputs=*//
  Selector1 : Selector  NumberOfDimensions=2  InputPortWidth=24  IndexOptions=Select all,Index vector (dialog)  Indices=1,1  OutputSizes=1,1
  Selector2 : Selector  NumberOfDimensions=2  InputPortWidth=24  IndexOptions=Select all,Index vector (dialog)  Indices=2,2  OutputSizes=1,1
  Selector3 : Selector  NumberOfDimensions=2  InputPortWidth=24  IndexOptions=Select all,Index vector (dialog)  Indices=3,3  OutputSizes=1,1
  Selector4 : Selector  NumberOfDimensions=2  InputPortWidth=24  IndexOptions=Select all,Index vector (dialog)  Indices=4,4  OutputSizes=1,1
  Selector5 : Selector  NumberOfDimensions=2  InputPortWidth=24  IndexOptions=Select all,Index vector (dialog)  Indices=5,5  OutputSizes=1,1
  Selector6 : Selector  NumberOfDimensions=2  InputPortWidth=24  IndexOptions=Select all,Index vector (dialog)  Indices=6,6  OutputSizes=1,1
  xk : ArgIn  DisableCoverage=on  OutDataTypeStr=single  PortDimensions=[NumModules*NumSeries,6]  ArgumentName=RC
  y : ArgOut  DisableCoverage=on  OutDataTypeStr=single  PortDimensions=[NumModules*NumSeries,NumberSt]  ArgumentName=F
  wires:
  Selector4/1 -> [C1]  "C1"
  Selector3/1 -> [R3]  "R3"
  Selector2/1 -> [R2]  "R2"
  Selector1/1 -> [R1]  "R1"
  Matrix Concatenate/1 -> y/1
  Exp/1 -> Matrix Concatenate/4
  Exp1/1 -> Matrix Concatenate/3
  Exp2/1 -> Matrix Concatenate/2
  Selector5/1 -> [C2]  "C2"
  Selector6/1 -> [C3]  "C3"
  Product/1 -> Exp1/1
  [R3] -> Product1/2
  [R2] -> Product/2
  [R1] -> Product2/2
  Product2/1 -> Exp2/1
  Constant1/1 -> Gain/1
  [C2] -> Product/3
  [C3] -> Product1/3
  Product1/1 -> Exp/1
  [C1] -> Product2/3
  Gain/1 -> Product1/1, Product/1, Product2/1
  xk/1 -> Selector4/1, Selector6/1, Selector5/1, Selector3/1, Selector2/1, Selector1/1
  Constant/1 -> Matrix Concatenate/1

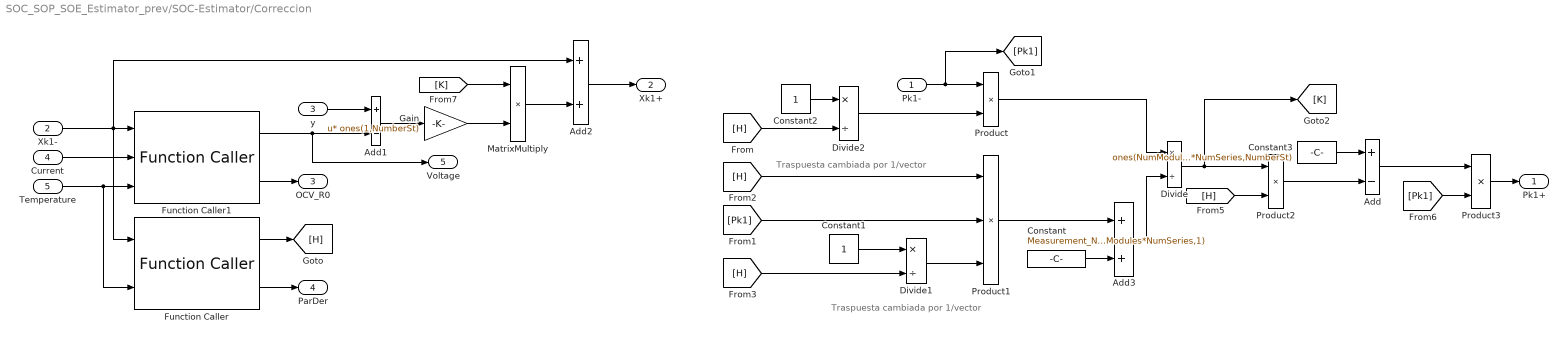
== system SOC_SOP_SOE_Estimator_prev/SOC-Estimator/Correccion ==
  note: Traspuesta cambiada por 1/vector
  note: Traspuesta cambiada por 1/vector
  Pk1- : Inport
  Xk1- : Inport  Port=2
  y : Inport  Port=3
  Current : Inport  Port=4
  Temperature : Inport  Port=5
  Add : Sum  Inputs=+-
  Add1 : Sum  Inputs=+-
  Add2 : Sum
  Add3 : Sum
  Constant : Constant  Value=Measurement_Noise_Covariance.*ones(NumModules*NumSeries,1)
  Constant1 : Constant  OutDataTypeStr=single
  Constant2 : Constant  OutDataTypeStr=single
  Constant3 : Constant  Value=ones(NumModules*NumSeries,NumberSt)  OutDataTypeStr=single
  Divide : Product  Inputs=*/
  Divide1 : Product  Inputs=*/
  Divide2 : Product  Inputs=*/
  Function Caller : FunctionCaller  FunctionPrototype=[H,ParDer] = observerJacobian2(xk,Temperature)  InputArgumentSpecifications=<Enter example>  OutputArgumentSpecifications=<Enter example>
  Function Caller1 : FunctionCaller  FunctionPrototype=[y,OCV_R0] = observer2(xk,Current,Temperature)  InputArgumentSpecifications=<Enter example>  OutputArgumentSpecifications=<Enter example>
  Gain : Gain  Gain=ones(1,NumberSt)  Multiplication=Matrix(u*K)
  MatrixMultiply : Product
  Product : Product
  Product1 : Product  Inputs=3
  Product2 : Product
  Product3 : Product
  Pk1+ : Outport
  Xk1+ : Outport  Port=2
  OCV_R0 : Outport  Port=3
  ParDer : Outport  Port=4
  Voltage : Outport  Port=5
  wires:
  Pk1-/1 -> [Pk1], Product/1
  Function Caller/1 -> [H]
  Divide2/1 -> Product/2
  Product/1 -> Divide/1
  [H] -> Product1/1
  [Pk1] -> Product1/2
  Divide1/1 -> Product1/3
  Product1/1 -> Add3/1
  Product2/1 -> Add/2
  [H] -> Product2/2
  Add/1 -> Product3/1
  [Pk1] -> Product3/2
  Product3/1 -> Pk1+/1
  y/1 -> Add1/1
  Function Caller1/1 -> Add1/2, Voltage/1
  MatrixMultiply/1 -> Add2/2
  Xk1-/1 -> Add2/1, Function Caller1/1, Function Caller/1
  Add2/1 -> Xk1+/1
  Add3/1 -> Divide/2
  Current/1 -> Function Caller1/2
  Temperature/1 -> Function Caller1/3, Function Caller/2
  Constant1/1 -> Divide1/1
  [H] -> Divide1/2
  [H] -> Divide2/2
  Constant2/1 -> Divide2/1
  Constant3/1 -> Add/1
  [K] -> MatrixMultiply/1
  Add1/1 -> Gain/1
  Gain/1 -> MatrixMultiply/2
  Function Caller1/2 -> OCV_R0/1
  Function Caller/2 -> ParDer/1
  Divide/1 -> [K], Product2/1
  Constant/1 -> Add3/2

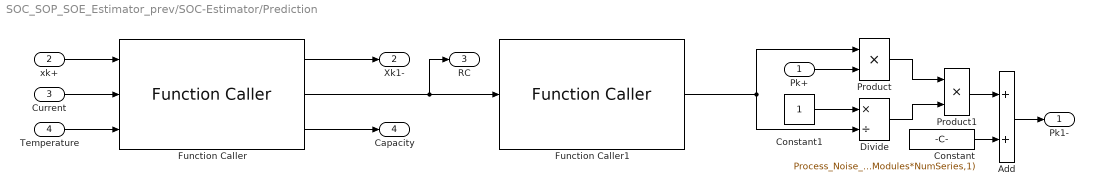
== system SOC_SOP_SOE_Estimator_prev/SOC-Estimator/Prediction ==
  Pk+ : Inport
  xk+ : Inport  Port=2
  Current : Inport  Port=3
  Temperature : Inport  Port=4
  Add : Sum
  Constant : Constant  Value=Process_Noise_Covariance.*ones(NumModules*NumSeries,1)
  Constant1 : Constant  OutDataTypeStr=single
  Divide : Product  Inputs=*/
  Function Caller : FunctionCaller  FunctionPrototype=[xk1,RC,Capacity] = state2(xk,Current,Temperature)  InputArgumentSpecifications=<Enter example>  OutputArgumentSpecifications=<Enter example>
  Function Caller1 : FunctionCaller  FunctionPrototype=F = stateJacobian2(RC)  InputArgumentSpecifications=<Enter example>  OutputArgumentSpecifications=<Enter example>
  Product : Product
  Product1 : Product
  Pk1- : Outport
  Xk1- : Outport  Port=2
  RC : Outport  Port=3
  Capacity : Outport  Port=4
  wires:
  Pk+/1 -> Product/2
  xk+/1 -> Function Caller/1
  Temperature/1 -> Function Caller/3
  Current/1 -> Function Caller/2
  Function Caller1/1 -> Product/1, Divide/2
  Divide/1 -> Product1/2
  Product/1 -> Product1/1
  Product1/1 -> Add/1
  Function Caller/1 -> Xk1-/1
  Add/1 -> Pk1-/1
  Constant1/1 -> Divide/1
  Function Caller/2 -> RC/1, Function Caller1/1
  Function Caller/3 -> Capacity/1
  Constant/1 -> Add/2

== matlab function SOC_SOP_SOE_Estimator_prev/SOP_Estimator/Max Current calculation ==
  data: V1 input; V2 input; V3 input; OCV input single; R0 input single; R1 input single; R2 input single; R3 input single; C1 input single; C2 input single; C3 input single; ParDer input; Ah input single; I_Max_Di output single; t input; L input; Vmin input; Vmax input; I_Max_Ch output single
function [I_Max_Di,I_Max_Ch] = fcn(V1,V2,V3,OCV,R0,R1,R2,R3,C1,C2,C3,ParDer,Ah,t,L,Vmin,Vmax)

% Temporal constants
tau1=R1.*C1;
tau2=R2.*C2;
tau3=R3.*C3;
% Equations
Numerator= OCV-V1.*exp((-L*t)./tau1)-V2.*exp((-L*t)./tau2)-V3.*exp((-L*t)./tau3);
Denominator= ((L*t./(Ah*3600)).*ParDer)+R0+R1.*(1-exp((-L*t)./tau1))+R2.*(1-exp((-L*t)./tau2))+R3.*(1-exp((-L*t)./tau3));

I_Max_Di = (Numerator-Vmin)./Denominator;

I_Max_Ch = (Numerator-Vmax)./Denominator;

== matlab function SOC_SOP_SOE_Estimator_prev/Simulink Function/x(k+1|k) calculation ==
  data: Ah input single; R1 input single; R2 input single; R3 input single; C1 input single; C2 input single; C3 input single; dx output single size=[NumSeries*NumModules,4]; V1 input single; V2 input single; V3 input single; current input single
function dx = fcn(Ah,R1,R2,R3,C1,C2,C3,V1,V2,V3,current)
l=length(R1);
dx = single(zeros(l,4));
% Cq is the battery capacity

dx(:,1) = -1./(Ah*3600)*current;
dx(:,2) = (1./C1)*current-V1./(R1.*C1);
dx(:,3) = (1./C2)*current-V2./(R2.*C2);
dx(:,4) = (1./C3)*current-V3./(R3.*C3);

== matlab function SOC_SOP_SOE_Estimator_prev/SOP_Estimator/Max Current calculation (SOC constraints) ==
  data: Ah input; I_Max_Di output; SOCmin input; SOCmax input; L input; Ts input; I_Max_Ch output; SOC input
function [I_Max_Di, I_Max_Ch]= fcn(Ah,SOCmin,SOCmax,L,Ts,SOC)

Numerator_dis= SOC-SOCmin;
Numerator_ch= SOC-SOCmax;
Denominator= (L*Ts)./(Ah*3600);

I_Max_Di = Numerator_dis./Denominator;

I_Max_Ch = Numerator_ch./Denominator;
